simulink model "error_at_arbitrary_input"  (R2021b)
settings: Solver=FixedStepAuto  StartTime=0.0  StopTime=100  FixedStep=0.01  RelTol=1e-3
libraries: simulink x2
settings Model: Creator=den  LastModifiedBy=den

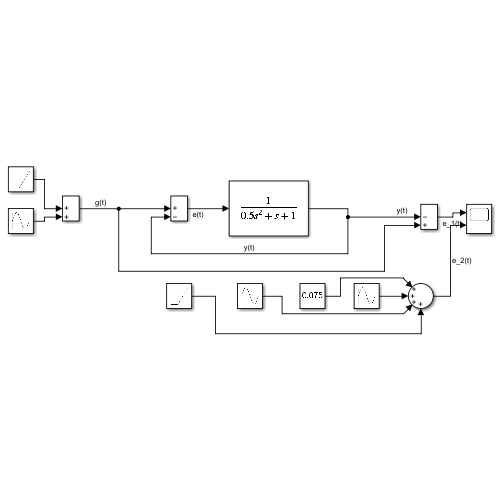
[thumbnail: Simulink's stored preview of the top-level diagram]
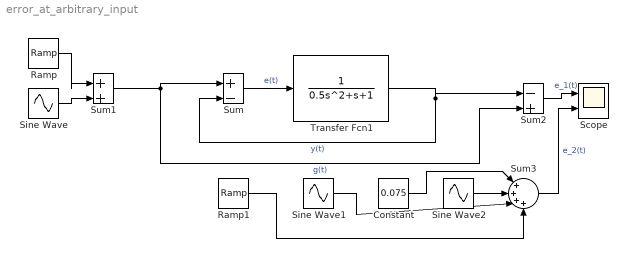
== system error_at_arbitrary_input ==
  Constant : Constant  Value=0.075
  Ramp : simulink/Sources/Ramp  slope=0.3  start=0  InitialOutput=0
  Ramp1 : simulink/Sources/Ramp  slope=0.15  start=0  InitialOutput=0
  Scope : Scope  NumInputPorts=2
  Sine Wave : Sin  Amplitude=2  Frequency=0.8  SampleTime=0
  Sine Wave1 : Sin  Frequency=0.8  SampleTime=0
  Sine Wave2 : Sin  Amplitude=0.464  Frequency=0.8  Phase=0.4*pi  SampleTime=0
  Sum : Sum  Inputs=|+-
  Sum1 : Sum  Inputs=|++
  Sum2 : Sum  Inputs=|-+
  Sum3 : Sum  Inputs=|++++
  Transfer Fcn1 : TransferFcn  Denominator=[0.5 1 1]
  wires:
  Transfer Fcn1/1 -> Sum2/1, Sum/2  "y(t)"
  Sum1/1 -> Sum2/2, Sum/1  "g(t)"
  Sine Wave/1 -> Sum1/2
  Ramp/1 -> Sum1/1
  Sum/1 -> Transfer Fcn1/1  "e(t)"
  Sum2/1 -> Scope/1  "e_1(t)"
  Sine Wave2/1 -> Sum3/2
  Constant/1 -> Sum3/1
  Sine Wave1/1 -> Sum3/3
  Ramp1/1 -> Sum3/4
  Sum3/1 -> Scope/2  "e_2(t)"
